simulink model "Slidingmode_Controller"  (R2016a)
settings: Solver=VariableStepAuto  StartTime=0.0  StopTime=200  FixedStep=1e-15  RelTol=1e-3
settings Model: Creator=Administrator  LastModifiedBy=Administrator

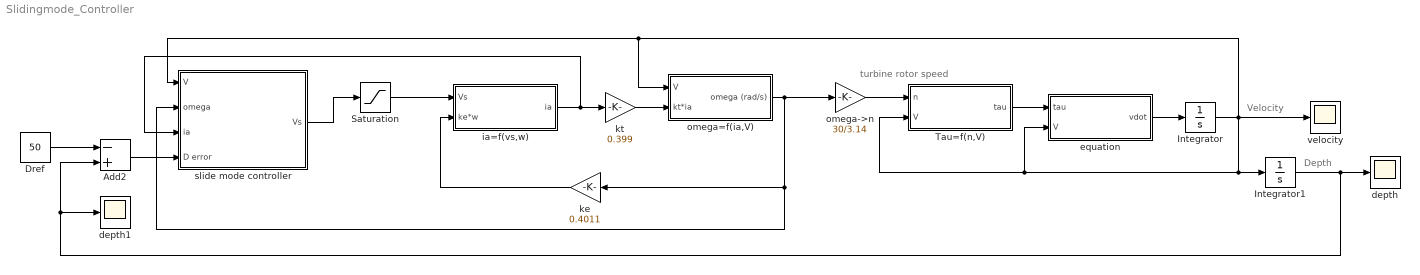
== system Slidingmode_Controller ==
  note: turbine rotor speed
  note: Depth
  note: Velocity
  Add2 : Sum  Inputs=-+
  Dref : Constant  Value=50
  Integrator : Integrator
  Integrator1 : Integrator
  Saturation : Saturate  UpperLimit=100  LowerLimit=-100
  Tau=f(n,V) : Subsystem
  depth : Scope
  depth1 : Scope
  equation : Subsystem
  ia=f(vs,w) : Subsystem
  ke : Gain  Gain=0.4011
  kt : Gain  Gain=0.399
  omega->n : Gain  Gain=30/3.14
  omega=f(ia,V) : Subsystem
  slide mode controller : Subsystem
  velocity : Scope
  wires:
  ia=f(vs,w)/1(ia) -> slide mode controller/3(ia), kt/1
  omega=f(ia,V)/1(omega (rad/s)) -> slide mode controller/2(omega), ke/1, omega->n/1
  ke/1 -> ia=f(vs,w)/2(ke*w)
  kt/1 -> omega=f(ia,V)/2(kt*ia)
  omega->n/1 -> Tau=f(n,V)/1(n)
  Tau=f(n,V)/1(tau) -> equation/1(tau)
  equation/1(vdot) -> Integrator/1
  Integrator/1 -> velocity/1, Integrator1/1, Tau=f(n,V)/2(V), equation/2(V), omega=f(ia,V)/1(V), slide mode controller/1(V)
  Integrator1/1 -> depth/1, depth1/1, Add2/2
  slide mode controller/1(Vs) -> Saturation/1
  Saturation/1 -> ia=f(vs,w)/1(Vs)
  Dref/1 -> Add2/1
  Add2/1 -> slide mode controller/4(D error)

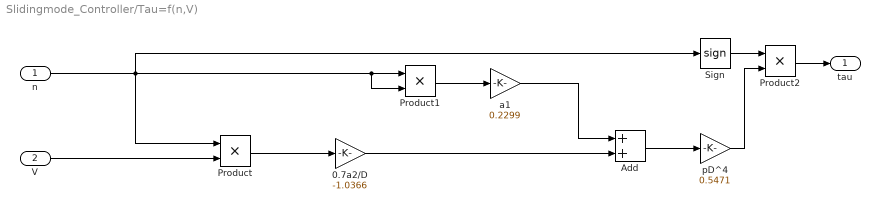
== system Slidingmode_Controller/Tau=f(n,V) ==
  n : Inport
  V : Inport  Port=2
  0.7a2/D : Gain  Gain=-1.0366
  Add : Sum
  Product : Product
  Product1 : Product
  Product2 : Product
  Sign : Signum
  a1 : Gain  Gain=0.2299
  pD^4 : Gain  Gain=0.5471
  tau : Outport
  wires:
  n/1 -> Sign/1, Product/1, Product1/2, Product1/1
  V/1 -> Product/2
  Product1/1 -> a1/1
  Product/1 -> 0.7a2/D/1
  a1/1 -> Add/1
  0.7a2/D/1 -> Add/2
  Add/1 -> pD^4/1
  Sign/1 -> Product2/1
  pD^4/1 -> Product2/2
  Product2/1 -> tau/1

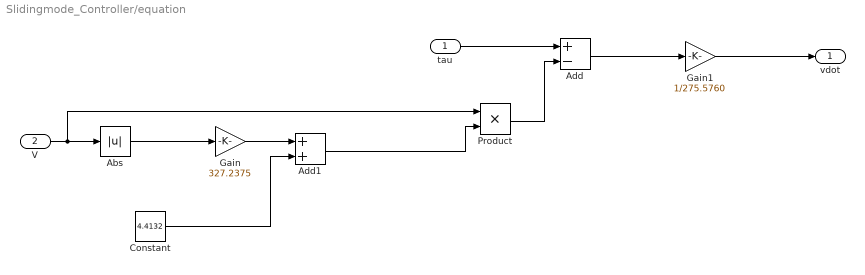
== system Slidingmode_Controller/equation ==
  tau : Inport
  V : Inport  Port=2
  Abs : Abs
  Add : Sum  Inputs=+-
  Add1 : Sum
  Constant : Constant  Value=4.4132
  Gain : Gain  Gain=327.2375
  Gain1 : Gain  Gain=1/275.5760
  Product : Product
  vdot : Outport
  wires:
  tau/1 -> Add/1
  V/1 -> Product/1, Abs/1
  Abs/1 -> Gain/1
  Gain/1 -> Add1/1
  Constant/1 -> Add1/2
  Add1/1 -> Product/2
  Product/1 -> Add/2
  Add/1 -> Gain1/1
  Gain1/1 -> vdot/1

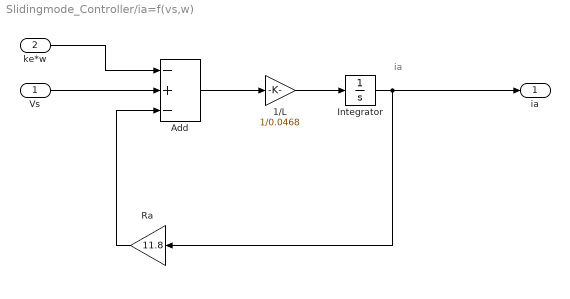
== system Slidingmode_Controller/ia=f(vs,w) ==
  note: ia
  Vs : Inport
  ke*w : Inport  Port=2
  1/L : Gain  Gain=1/0.0468
  Add : Sum  Inputs=-+-
  Integrator : Integrator
  Ra : Gain  Gain=11.8
  ia : Outport
  wires:
  Add/1 -> 1/L/1
  1/L/1 -> Integrator/1
  Integrator/1 -> ia/1, Ra/1
  Ra/1 -> Add/3
  Vs/1 -> Add/2
  ke*w/1 -> Add/1

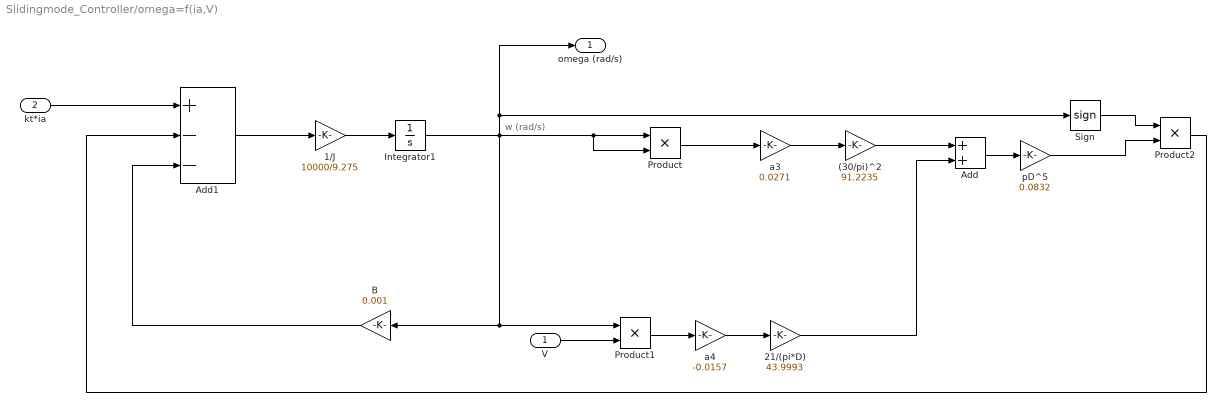
== system Slidingmode_Controller/omega=f(ia,V) ==
  note: w (rad/s)
  V : Inport
  kt*ia : Inport  Port=2
  (30/pi)^2 : Gain  Gain=91.2235
  1/J : Gain  Gain=10000/9.275
  21/(pi*D) : Gain  Gain=43.9993
  Add : Sum
  Add1 : Sum  Inputs=+--
  B : Gain  Gain=0.001
  Integrator1 : Integrator
  Product : Product
  Product1 : Product
  Product2 : Product
  Sign : Signum
  a3 : Gain  Gain=0.0271
  a4 : Gain  Gain=-0.0157
  pD^5 : Gain  Gain=0.0832
  omega (rad/s) : Outport
  wires:
  1/J/1 -> Integrator1/1
  Add1/1 -> 1/J/1
  B/1 -> Add1/3
  Integrator1/1 -> Product/2, Product/1, omega (rad/s)/1, Sign/1, Product1/1, B/1
  kt*ia/1 -> Add1/1
  Product/1 -> a3/1
  a3/1 -> (30/pi)^2/1
  (30/pi)^2/1 -> Add/1
  a4/1 -> 21/(pi*D)/1
  V/1 -> Product1/2
  Product1/1 -> a4/1
  21/(pi*D)/1 -> Add/2
  Add/1 -> pD^5/1
  Sign/1 -> Product2/1
  pD^5/1 -> Product2/2
  Product2/1 -> Add1/2

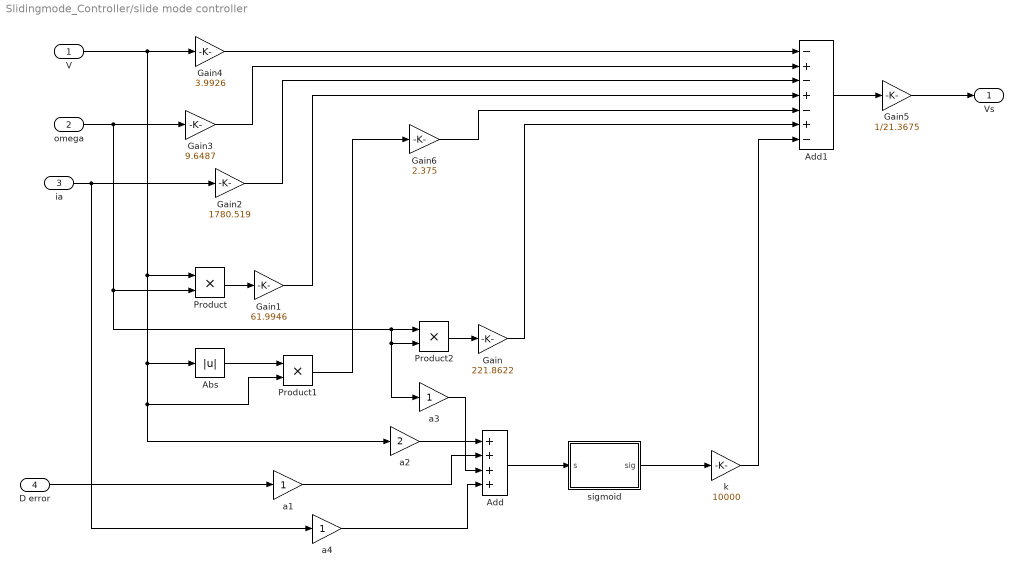
== system Slidingmode_Controller/slide mode controller ==
  V : Inport
  omega : Inport  Port=2
  ia : Inport  Port=3
  D error : Inport  Port=4
  Abs : Abs
  Add : Sum  Inputs=++++
  Add1 : Sum  Inputs=-+-+-+-
  Gain : Gain  Gain=221.8622
  Gain1 : Gain  Gain=61.9946
  Gain2 : Gain  Gain=1780.519
  Gain3 : Gain  Gain=9.6487
  Gain4 : Gain  Gain=3.9926
  Gain5 : Gain  Gain=1/21.3675
  Gain6 : Gain  Gain=2.375
  Product : Product
  Product1 : Product
  Product2 : Product
  a1 : Gain
  a2 : Gain  Gain=2
  a3 : Gain
  a4 : Gain
  k : Gain  Gain=10000
  sigmoid : MATLAB Function  TreatAsAtomicUnit=on
  Vs : Outport
  wires:
  V/1 -> a2/1, Product1/2, Abs/1, Product/1, Gain4/1
  omega/1 -> a3/1, Product2/2, Product2/1, Product/2, Gain3/1
  ia/1 -> a4/1, Gain2/1
  Product/1 -> Gain1/1
  Gain4/1 -> Add1/1
  Gain3/1 -> Add1/2
  Gain2/1 -> Add1/3
  Gain1/1 -> Add1/4
  Abs/1 -> Product1/1
  Product2/1 -> Gain/1
  Gain/1 -> Add1/6
  D error/1 -> a1/1
  a2/1 -> Add/1
  a1/1 -> Add/2
  k/1 -> Add1/7
  Add1/1 -> Gain5/1
  Gain5/1 -> Vs/1
  a4/1 -> Add/4
  Add/1 -> sigmoid/1(s)
  Gain6/1 -> Add1/5
  Product1/1 -> Gain6/1
  sigmoid/1(sig) -> k/1
  a3/1 -> Add/3

== matlab function Slidingmode_Controller/slide mode controller/sigmoid ==
  data: s input; sig output
function sig = fcn(s)
%#codegen
if s<=-1
    u=-1;
else if s>-1&&s<=1
        u=s;
    else
        u=1;
    end
end        

sig = u;
